simulink model "quadsim_sol"  (R2019a)
settings: Solver=ode45  StartTime=0.0  StopTime=20  FixedStep=0.001  RelTol=1e-3  EnableMultiTasking=on
InitFcn:
  | param
undefined symbols (not defined in the file or in its folder): controller, P, trajectory
settings Model: NumberOfSteps=100  Creator=ecestudent  LastModifiedBy=USER
settings DataIOCC: LimitDataPoints=on  SaveFormat=Array  ReturnWorkspaceOutputs=off
settings OptimizationCC: LifeSpan=inf
settings DebuggingCC: SFUnexpectedBacktrackingDiag=warning  SFNoUnconditionalDefaultTransitionDiag=warning  SFExecutionAtInitializationDiag=none  ArithmeticOperatorsInVariantConditions=warning
settings HardwareCC: ProdBitPerPointer=32  ProdBitPerSizeT=32  ProdBitPerPtrDiffT=32  ProdLargestAtomicFloat=None  ProdIntDivRoundTo=Undefined  ProdEndianess=Unspecified  ProdWordSize=32  ProdHWDeviceType=32-bit Generic
settings ModelReferenceCC: PropagateSignalLabelsOutOfModel=off
settings SFSimCC: SimUseLocalCustomCode=off
settings RTWCC: RTWUseLocalCustomCode=off
settings CodeAppCC: StateflowObjectComments=on
settings GRTTargetCC: TargetLangStandard=C89/C90 (ANSI)  GeneratePreprocessorConditionals=Disable all
settings ConfigComp: CovMetricSettings=dw  CovHtmlReporting=on  CovSaveCumulativeToWorkspaceVar=on  CovSaveSingleToWorkspaceVar=on  CovExternalEMLEnable=off
settings SimscapeCC: SimscapeNormalizeSystem=off

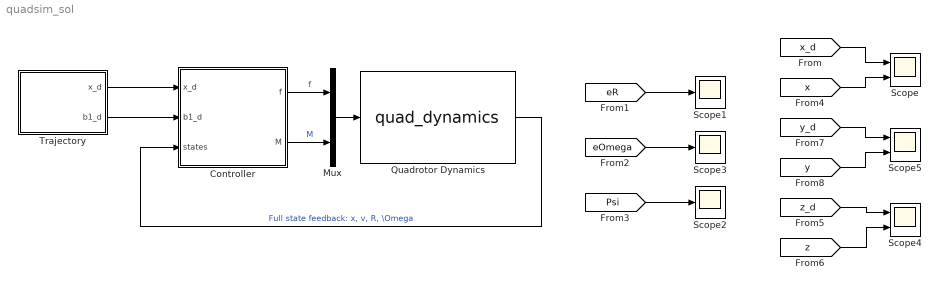
== system quadsim_sol ==
  Controller : Subsystem
  Mux : Mux  Inputs=2
  Quadrotor Dynamics : S-Function  FunctionName=quad_dynamics  Parameters=P  SFunctionDeploymentMode=off  EnableBusSupport=off
  Scope : Scope  NumInputPorts=2
  Scope1 : Scope
  Scope2 : Scope
  Scope3 : Scope
  Scope4 : Scope  NumInputPorts=2
  Scope5 : Scope  NumInputPorts=2
  Trajectory : Subsystem
  wires:
  Mux/1 -> Quadrotor Dynamics/1
  Quadrotor Dynamics/1 -> Controller/3(states)  "Full state feedback: x, v, R, \\Omega"
  Controller/1(f) -> Mux/1  "f"
  Controller/2(M) -> Mux/2  "M"
  Trajectory/1(x_d) -> Controller/1(x_d)
  Trajectory/2(b1_d) -> Controller/2(b1_d)
  [eR] -> Scope1/1
  [eOmega] -> Scope3/1
  [Psi] -> Scope2/1
  [x_d] -> Scope/1
  [x] -> Scope/2
  [z] -> Scope4/2
  [z_d] -> Scope4/1
  [y] -> Scope5/2
  [y_d] -> Scope5/1

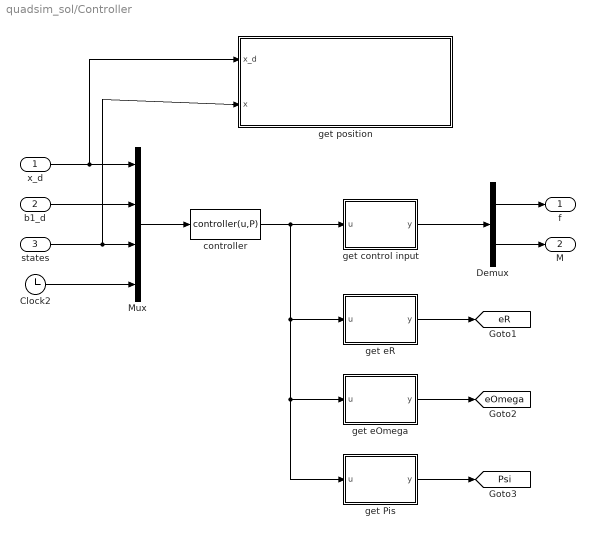
== system quadsim_sol/Controller ==
  x_d : Inport
  b1_d : Inport  Port=2
  states : Inport  Port=3
  Clock2 : Clock
  Demux : Demux  Outputs=2
  Mux : Mux
  controller : MATLABFcn  MATLABFcn=controller(u,P)  OutputDimensions=11  SampleTime=P.Ts
  get Pis : MATLAB Function  TreatAsAtomicUnit=on
  get control input : MATLAB Function  TreatAsAtomicUnit=on
  get eOmega : MATLAB Function  TreatAsAtomicUnit=on
  get eR : MATLAB Function  TreatAsAtomicUnit=on
  get position : Subsystem
  f : Outport
  M : Outport  Port=2
  tag scope: Psi=global, eOmega=global, eR=global
  wires:
  Clock2/1 -> Mux/4
  Mux/1 -> controller/1
  x_d/1 -> get position/1(x_d), Mux/1
  states/1 -> get position/2(x), Mux/3
  Demux/1 -> f/1
  Demux/2 -> M/1
  b1_d/1 -> Mux/2
  controller/1 -> get Pis/1(u), get eOmega/1(u), get eR/1(u), get control input/1(u)
  get eR/1(y) -> [eR]
  get eOmega/1(y) -> [eOmega]
  get control input/1(y) -> Demux/1
  get Pis/1(y) -> [Psi]

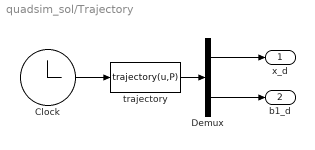
== system quadsim_sol/Trajectory ==
  Clock : Clock
  Demux : Demux  Outputs=2
  trajectory : MATLABFcn  MATLABFcn=trajectory(u,P)  OutputDimensions=12
  x_d : Outport
  b1_d : Outport  Port=2
  wires:
  Clock/1 -> trajectory/1
  trajectory/1 -> Demux/1
  Demux/1 -> x_d/1
  Demux/2 -> b1_d/1

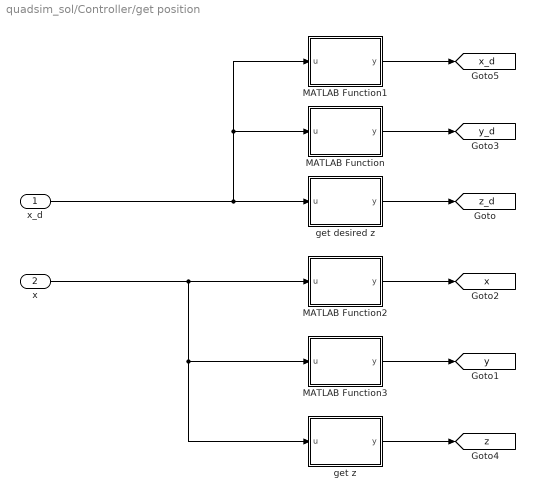
== system quadsim_sol/Controller/get position ==
  x_d : Inport
  x : Inport  Port=2
  MATLAB Function : MATLAB Function  TreatAsAtomicUnit=on
  MATLAB Function1 : MATLAB Function  TreatAsAtomicUnit=on
  MATLAB Function2 : MATLAB Function  TreatAsAtomicUnit=on
  MATLAB Function3 : MATLAB Function  TreatAsAtomicUnit=on
  get desired z : MATLAB Function  TreatAsAtomicUnit=on
  get z : MATLAB Function  TreatAsAtomicUnit=on
  tag scope: x=global, x_d=global, y=global, y_d=global, z=global, z_d=global
  wires:
  get desired z/1(y) -> [z_d]
  get z/1(y) -> [z]
  x_d/1 -> MATLAB Function1/1(u), MATLAB Function/1(u), get desired z/1(u)
  x/1 -> MATLAB Function2/1(u), MATLAB Function3/1(u), get z/1(u)
  MATLAB Function2/1(y) -> [x]
  MATLAB Function3/1(y) -> [y]
  MATLAB Function1/1(y) -> [x_d]
  MATLAB Function/1(y) -> [y_d]

== matlab function quadsim_sol/Controller/get eR ==
  data: u input; y output
function y = fcn(u)

y = u(5:7);

== matlab function quadsim_sol/Controller/get position/get desired z ==
  data: u input; y output
function y = fcn(u)

y = u(3);

== matlab function quadsim_sol/Controller/get eOmega ==
  data: u input; y output
function y = fcn(u)

y = u(8:10);

== matlab function quadsim_sol/Controller/get control input ==
  data: u input; y output
function y = fcn(u)

y = u(1:4);

== matlab function quadsim_sol/Controller/get Pis ==
  data: u input; y output
function y = fcn(u)

y = u(11);

== matlab function quadsim_sol/Controller/get position/get z ==
  data: u input; y output
function y = fcn(u)

y = u(3);

== matlab function quadsim_sol/Controller/get position/MATLAB Function ==
  data: u input; y output
function y = fcn(u)

y = u(2);

== matlab function quadsim_sol/Controller/get position/MATLAB Function1 ==
  data: u input; y output
function y = fcn(u)

y = u(1);

== matlab function quadsim_sol/Controller/get position/MATLAB Function2 ==
  data: u input; y output
function y = fcn(u)

y = u(1);

== matlab function quadsim_sol/Controller/get position/MATLAB Function3 ==
  data: u input; y output
function y = fcn(u)

y = u(2);
